simulink model "q3__inductor"  (R2018a)
settings: Solver=FixedStepDiscrete  StartTime=0.0  StopTime=0.06  FixedStep=1e-6  RelTol=1e-3
libraries: powerlib x16
settings Model: Creator=burya  LastModifiedBy=burya

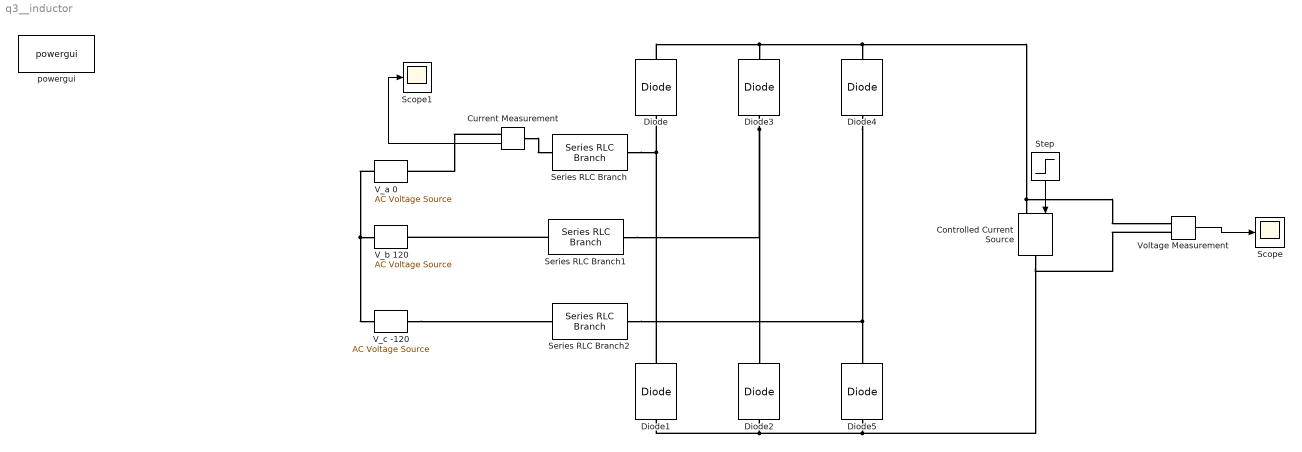
== system q3__inductor ==
  Controlled Current Source : powerlib/Electrical Sources/Controlled Current Source  Initialize=on  Source_Type=DC  Amplitude=40  Phase=0  Frequency=0  Measurements=None
  Current Measurement : powerlib/Measurements/Current Measurement  PhasorSimulation=off  OutputType=Complex  PSBequivalent=0
  Diode{,1..5} (6 alike) : powerlib/Power Electronics/Diode  Ron=1e-9  Lon=0  Vf=0  IC=0  UseSnubber=0  Rs=500  Cs=250e-9  Measurements=off
  Scope : Scope
  Scope1 : Scope
  Series RLC Branch : powerlib/Elements/Series RLC Branch  LConnTagsString=__new0  RConnTagsString=__new0  BranchType=L  Resistance=1  Inductance=1e-3  SetiL0=off  InitialCurrent=1.103  Capacitance=1e-6  Setx0=off  InitialVoltage=0  Measurements=None
  Series RLC Branch1 : powerlib/Elements/Series RLC Branch  LConnTagsString=__new0  RConnTagsString=__new0  BranchType=L  Resistance=1  Inductance=1e-3  SetiL0=off  InitialCurrent=0  Capacitance=1e-6  Setx0=off  InitialVoltage=0  Measurements=None
  Series RLC Branch2 : powerlib/Elements/Series RLC Branch  LConnTagsString=__new0  RConnTagsString=__new0  BranchType=L  Resistance=1  Inductance=1e-3  SetiL0=off  InitialCurrent=0  Capacitance=1e-6  Setx0=off  InitialVoltage=0  Measurements=None
  Step : Step  Time=0  SampleTime=1e-6
  "V_a 0 " : powerlib/Electrical Sources/AC Voltage Source  Amplitude=230*sqrt(2)  Phase=0  Frequency=50  SampleTime=1e-6  Measurements=None  BusType=swing  Pref=10e3  Qref=0  Qmin=-inf  Qmax=+inf
  "V_b 120 " : powerlib/Electrical Sources/AC Voltage Source  Amplitude=230*sqrt(2)  Phase=120  Frequency=50  SampleTime=1e-6  Measurements=None  BusType=swing  Pref=10e3  Qref=0  Qmin=-inf  Qmax=+inf
  "V_c -120 " : powerlib/Electrical Sources/AC Voltage Source  Amplitude=230*sqrt(2)  Phase=-120  Frequency=50  SampleTime=1e-6  Measurements=None  BusType=swing  Pref=10e3  Qref=0  Qmin=-inf  Qmax=+inf
  Voltage Measurement : powerlib/Measurements/Voltage Measurement  PhasorSimulation=off  OutputType=Complex  PSBequivalent=0
  powergui : powerlib/powergui  Priority=1  SimulationMode=Discrete  SampleTime=1e-6  frequency=60  Iterations=50  frequencyindice=50  Pbase=100e6  ErrMax=1e-4  UnitsV=kV  UnitsW=MW  buscounter=0  FunctionMessages=off  echomessages=off  EnableUseOfTLC=off  CurrentSourceSwitches=off  DisableSnubberDevices=off  DisableRonSwitches=off  DisableVfSwitches=off  DisplayEquations=off  SolverType=Tustin/Backward Euler (TBE)  Interpol=off  ExternalGateDelay=off  methode=off  Ts=100  x0status=blocks  SPID=on  SwTol=0  HookPort=off  RestoreLinks=warning  ResistiveCurrentMeasurement=off  Frange=[0:2:500]  Ylog=off  Xlog=on  ShowGrid=off  save=off  variable=ZData  structure=input_current_a  ZoomFFT=off  StartTime=0.01  cycles=12  DisplayStyle=1  fundamental=300  FreqAxis=off  MaxFrequency=9000  frequencyindicesteady=1  RmsSteady=1  display=off
  wires:
  Voltage Measurement/1 -> Scope/1
  Current Measurement/1 -> Scope1/1
  Step/1 -> Controlled Current Source/1
  connections:
  Current Measurement/LConn1 -- Series RLC Branch/LConn1
  Diode/RConn1 -- Voltage Measurement/LConn1 -- Controlled Current Source/LConn1 -- Diode4/RConn1 -- Diode3/RConn1
  Diode4/LConn1 -- Series RLC Branch2/RConn1 -- Diode5/RConn1
  Diode5/LConn1 -- Voltage Measurement/LConn2 -- Controlled Current Source/RConn1 -- Diode1/LConn1 -- Diode2/LConn1
  "V_a 0 "/LConn1 -- "V_c -120 "/LConn1 -- "V_b 120 "/LConn1
  Diode3/LConn1 -- Series RLC Branch1/RConn1 -- Diode2/RConn1
  Current Measurement/RConn1 -- "V_a 0 "/RConn1
  Series RLC Branch/RConn1 -- Diode1/RConn1 -- Diode/LConn1
  Series RLC Branch1/LConn1 -- "V_b 120 "/RConn1
  "V_c -120 "/RConn1 -- Series RLC Branch2/LConn1
